simulink model "Copy_of_signal_injection"  (R2023a)
settings: Solver=FixedStepAuto  StartTime=0.0  StopTime=1/(f_fund)/6  FixedStep=1e-7  RelTol=1e-3
InitFcn:
  | f_fund=50;
  | ma=1;
  | fsw=100e3;
settings Model: Creator=enesa  LastModifiedBy=enesa

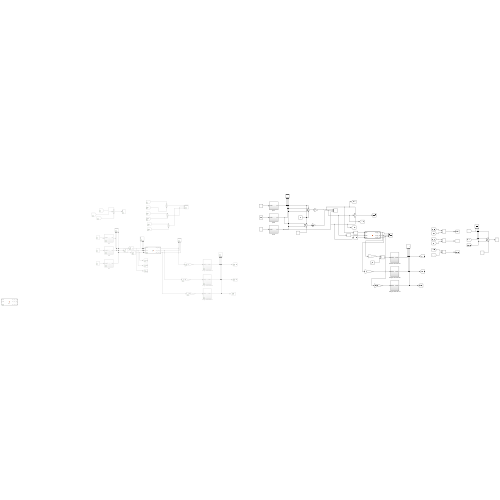
[thumbnail: Simulink's stored preview of the top-level diagram]
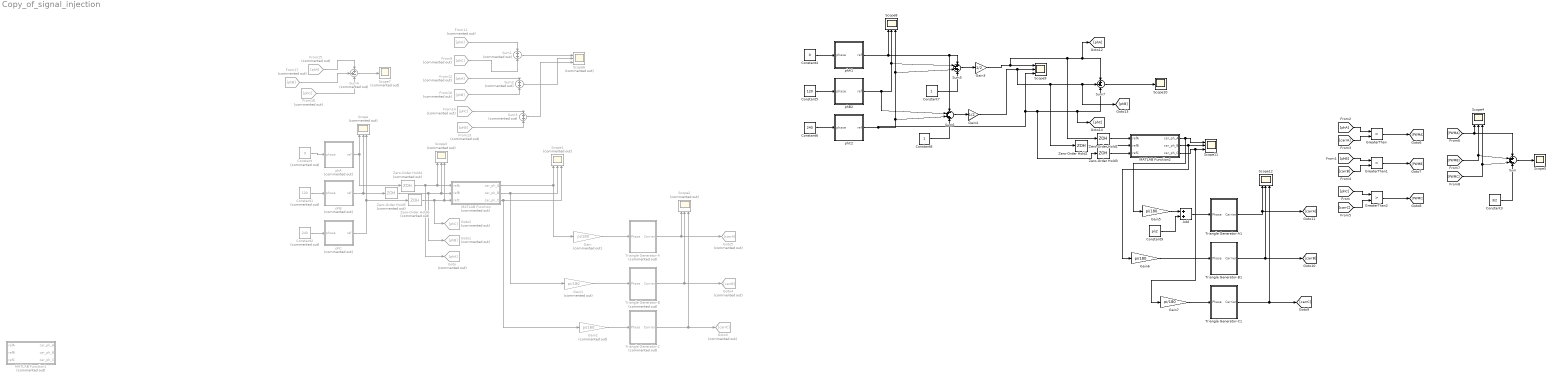
== system Copy_of_signal_injection ==
  Add : Sum
  Constant : Constant  Commented=on  Value=0
  Constant1 : Constant  Commented=on  Value=120
  Constant2 : Constant  Commented=on  Value=240
  Constant3 : Constant  Value=3/2
  Constant4 : Constant  Value=0
  Constant5 : Constant  Value=120
  Constant6 : Constant  Value=240
  Constant7 : Constant
  Constant8 : Constant
  Constant9 : Constant  Value=pi\2
  From10 : From  Commented=on  GotoTag=phB
  From11 : From  Commented=on  GotoTag=phA
  From12 : From  Commented=on  GotoTag=phA
  From13 : From  Commented=on  GotoTag=phB
  From14 : From  Commented=on  GotoTag=phC
  From15 : From  Commented=on  GotoTag=phA
  From16 : From  Commented=on  GotoTag=phC
  From17 : From  Commented=on  GotoTag=phB
  From9 : From  Commented=on  GotoTag=phC
  Gain : Gain  Commented=on  Gain=pi/180
  Gain1 : Gain  Commented=on  Gain=pi/180
  Gain2 : Gain  Commented=on  Gain=pi/180
  Gain3 : Gain  Gain=1/2
  Gain4 : Gain  Gain=1/2
  Gain5 : Gain  Gain=pi/180
  Gain6 : Gain  Gain=pi/180
  Gain7 : Gain  Gain=pi/180
  Goto : Goto  Commented=on  GotoTag=phA
  Goto1 : Goto  Commented=on  GotoTag=phB
  Goto2 : Goto  Commented=on  GotoTag=phC
  Goto3 : Goto  Commented=on  GotoTag=carrC
  Goto4 : Goto  Commented=on  GotoTag=carrB
  Goto5 : Goto  Commented=on  GotoTag=carrA
  GreaterThan : RelationalOperator  Operator=>  OutDataTypeStr=boolean  RndMeth=Simplest  InputSameDT=off
  GreaterThan1 : RelationalOperator  Operator=>  OutDataTypeStr=boolean  RndMeth=Simplest  InputSameDT=off
  GreaterThan2 : RelationalOperator  Operator=>  OutDataTypeStr=boolean  RndMeth=Simplest  InputSameDT=off
  MATLAB Function : MATLAB Function  Commented=on  TreatAsAtomicUnit=on
  MATLAB Function1 : MATLAB Function  Commented=on  TreatAsAtomicUnit=on
  MATLAB Function2 : MATLAB Function  TreatAsAtomicUnit=on
  Scope{,1..3,6} (5 alike) : Scope  Commented=on  NumInputPorts=3
  Scope10 : Scope
  Scope{4,8..9,11..12} (5 alike) : Scope  NumInputPorts=3
  Scope5 : Scope
  Scope7 : Scope  Commented=on
  Sum : Sum  Inputs=+++-
  Sum1 : Sum  Commented=on
  Sum2 : Sum  Commented=on
  Sum3 : Sum  Commented=on
  Sum4 : Sum  Commented=on  Inputs=++-
  Sum5 : Sum  Inputs=+-++
  Sum6 : Sum  Inputs=-+++
  Sum7 : Sum  Inputs=++-
  Triangle Generator-A : Subsystem  Commented=on
  Triangle Generator-A1 : Subsystem
  Triangle Generator-B : Subsystem  Commented=on
  Triangle Generator-B1 : Subsystem
  Triangle Generator-C : Subsystem  Commented=on
  Triangle Generator-C1 : Subsystem
  Zero-Order Hold1 : ZeroOrderHold  SampleTime=20/fsw
  Zero-Order Hold2 : ZeroOrderHold  SampleTime=20/fsw
  Zero-Order Hold3 : ZeroOrderHold  SampleTime=20/fsw
  Zero-Order Hold4 : ZeroOrderHold  Commented=on  SampleTime=20/fsw
  Zero-Order Hold5 : ZeroOrderHold  Commented=on  SampleTime=20/fsw
  Zero-Order Hold6 : ZeroOrderHold  Commented=on  SampleTime=20/fsw
  phA : Subsystem  Commented=on
  phA1 : Subsystem
  phB : Subsystem  Commented=on
  phB2 : Subsystem
  phC : Subsystem  Commented=on
  phC2 : Subsystem
  wires:
  Constant/1 -> phA/1(phase)
  Constant1/1 -> phB/1(phase)
  Constant2/1 -> phC/1(phase)
  phA/1(ref) -> Scope/1, Zero-Order Hold4/1
  phB/1(ref) -> Scope/2, Zero-Order Hold5/1
  phC/1(ref) -> Scope/3, Zero-Order Hold6/1
  MATLAB Function/1(car_ph_A) -> Gain/1, Scope1/1
  MATLAB Function/3(car_ph_C) -> Gain2/1, Scope1/3
  MATLAB Function/2(car_ph_B) -> Gain1/1, Scope1/2
  Triangle Generator-B/1(Carrier) -> Goto4/1, Scope2/2
  Triangle Generator-C/1(Carrier) -> Goto3/1, Scope2/3
  Zero-Order Hold4/1 -> Scope3/1, MATLAB Function/1(refA), Goto/1
  Zero-Order Hold5/1 -> Goto1/1, Scope3/2, MATLAB Function/2(refB)
  Zero-Order Hold6/1 -> Goto2/1, Scope3/3, MATLAB Function/3(refC)
  Triangle Generator-A/1(Carrier) -> Goto5/1, Scope2/1
  [phA] -> GreaterThan/1
  [carrA] -> GreaterThan/2
  [phB] -> GreaterThan1/1
  [carrB] -> GreaterThan1/2
  [phC] -> GreaterThan2/1
  [carrC] -> GreaterThan2/2
  GreaterThan/1 -> [PWMA]
  GreaterThan1/1 -> [PWMB]
  GreaterThan2/1 -> [PWMC]
  [PWMA] -> Sum/1, Scope4/1
  [PWMB] -> Sum/2, Scope4/2
  [PWMC] -> Sum/3, Scope4/3
  Gain/1 -> Triangle Generator-A/1(Phase)
  Gain1/1 -> Triangle Generator-B/1(Phase)
  Gain2/1 -> Triangle Generator-C/1(Phase)
  Sum/1 -> Scope5/1
  Constant3/1 -> Sum/4
  From11/1 -> Sum1/1
  From9/1 -> Sum1/2
  Sum1/1 -> Scope6/1
  From12/1 -> Sum2/1
  From10/1 -> Sum2/2
  Sum2/1 -> Scope6/2
  From13/1 -> Sum3/2
  From14/1 -> Sum3/1
  Sum3/1 -> Scope6/3
  From15/1 -> Sum4/1
  From16/1 -> Sum4/3
  From17/1 -> Sum4/2
  Sum4/1 -> Scope7/1
  Constant6/1 -> phC2/1(phase)
  Constant4/1 -> phA1/1(phase)
  Constant5/1 -> phB2/1(phase)
  Constant7/1 -> Sum5/4
  Sum5/1 -> Gain3/1
  phA1/1(ref) -> Sum6/1, Sum5/1, Scope8/1
  Constant8/1 -> Sum6/4
  Sum6/1 -> Gain4/1
  phB2/1(ref) -> Sum6/2, Sum5/2, Scope8/2
  Gain4/1 -> Zero-Order Hold2/1, [phB], Sum7/2, Scope9/2
  Sum7/1 -> Scope10/1
  MATLAB Function2/1(car_ph_A) -> Gain5/1, Scope11/1
  MATLAB Function2/2(car_ph_B) -> Gain6/1, Scope11/2
  MATLAB Function2/3(car_ph_C) -> Gain7/1, Scope11/3
  phC2/1(ref) -> Zero-Order Hold3/1, [phC], Sum7/3, Scope9/3, Sum6/3, Sum5/3, Scope8/3
  Triangle Generator-A1/1(Carrier) -> [carrA], Scope12/1
  Gain7/1 -> Triangle Generator-C1/1(Phase)
  Gain6/1 -> Triangle Generator-B1/1(Phase)
  Gain3/1 -> [phA], Sum7/1, Zero-Order Hold1/1, Scope9/1
  Triangle Generator-B1/1(Carrier) -> [carrB], Scope12/2
  Triangle Generator-C1/1(Carrier) -> [carrC], Scope12/3
  Zero-Order Hold1/1 -> MATLAB Function2/1(refA)
  Zero-Order Hold2/1 -> MATLAB Function2/2(refB)
  Zero-Order Hold3/1 -> MATLAB Function2/3(refC)
  Gain5/1 -> Add/1
  Constant9/1 -> Add/2
  Add/1 -> Triangle Generator-A1/1(Phase)

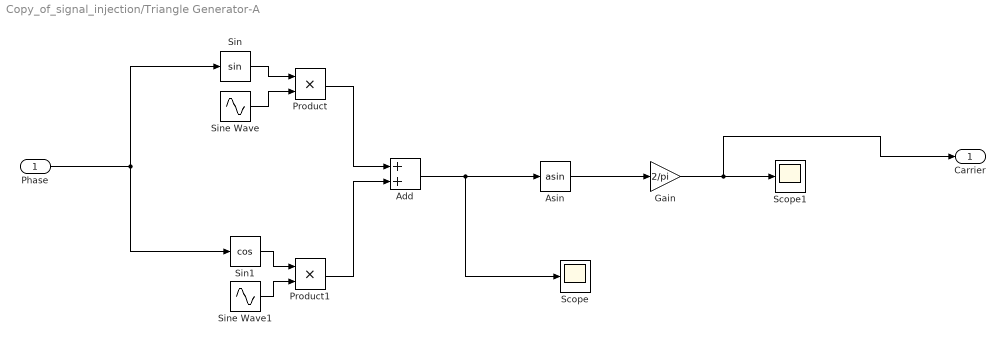
== system Copy_of_signal_injection/Triangle Generator-A ==
  Phase : Inport
  Add : Sum
  Asin : Trigonometry  Operator=asin
  Gain : Gain  Gain=2/pi
  Product : Product
  Product1 : Product
  Scope : Scope
  Scope1 : Scope
  Sin : Trigonometry
  Sin1 : Trigonometry  Operator=cos
  Sine Wave : Sin  Frequency=2*pi*fsw  SampleTime=0
  Sine Wave1 : Sin  Frequency=2*pi*fsw  Phase=-pi/2  SampleTime=0
  Carrier : Outport
  wires:
  Sin/1 -> Product/1
  Sine Wave/1 -> Product/2
  Phase/1 -> Sin/1, Sin1/1
  Product/1 -> Add/1
  Asin/1 -> Gain/1
  Gain/1 -> Carrier/1, Scope1/1
  Sine Wave1/1 -> Product1/2
  Product1/1 -> Add/2
  Add/1 -> Asin/1, Scope/1
  Sin1/1 -> Product1/1

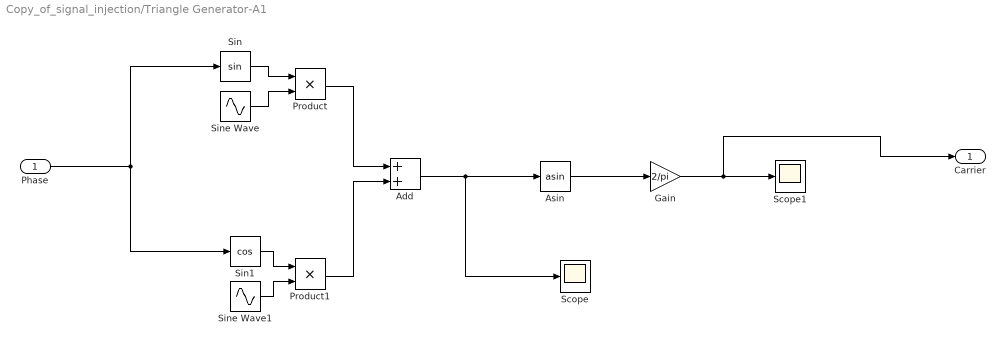
== system Copy_of_signal_injection/Triangle Generator-A1 ==
  Phase : Inport
  Add : Sum
  Asin : Trigonometry  Operator=asin
  Gain : Gain  Gain=2/pi
  Product : Product
  Product1 : Product
  Scope : Scope
  Scope1 : Scope
  Sin : Trigonometry
  Sin1 : Trigonometry  Operator=cos
  Sine Wave : Sin  Frequency=2*pi*fsw  SampleTime=0
  Sine Wave1 : Sin  Frequency=2*pi*fsw  Phase=-pi/2  SampleTime=0
  Carrier : Outport
  wires:
  Sin/1 -> Product/1
  Sine Wave/1 -> Product/2
  Phase/1 -> Sin/1, Sin1/1
  Product/1 -> Add/1
  Asin/1 -> Gain/1
  Gain/1 -> Carrier/1, Scope1/1
  Sine Wave1/1 -> Product1/2
  Product1/1 -> Add/2
  Add/1 -> Asin/1, Scope/1
  Sin1/1 -> Product1/1

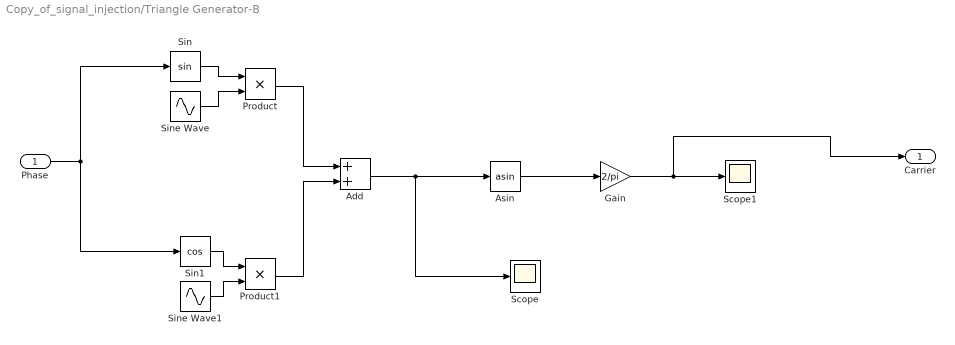
== system Copy_of_signal_injection/Triangle Generator-B ==
  Phase : Inport
  Add : Sum
  Asin : Trigonometry  Operator=asin
  Gain : Gain  Gain=2/pi
  Product : Product
  Product1 : Product
  Scope : Scope
  Scope1 : Scope
  Sin : Trigonometry
  Sin1 : Trigonometry  Operator=cos
  Sine Wave : Sin  Frequency=2*pi*fsw  SampleTime=0
  Sine Wave1 : Sin  Frequency=2*pi*fsw  Phase=-pi/2  SampleTime=0
  Carrier : Outport
  wires:
  Sin/1 -> Product/1
  Sine Wave/1 -> Product/2
  Phase/1 -> Sin1/1, Sin/1
  Product/1 -> Add/1
  Asin/1 -> Gain/1
  Gain/1 -> Carrier/1, Scope1/1
  Sine Wave1/1 -> Product1/2
  Product1/1 -> Add/2
  Add/1 -> Asin/1, Scope/1
  Sin1/1 -> Product1/1

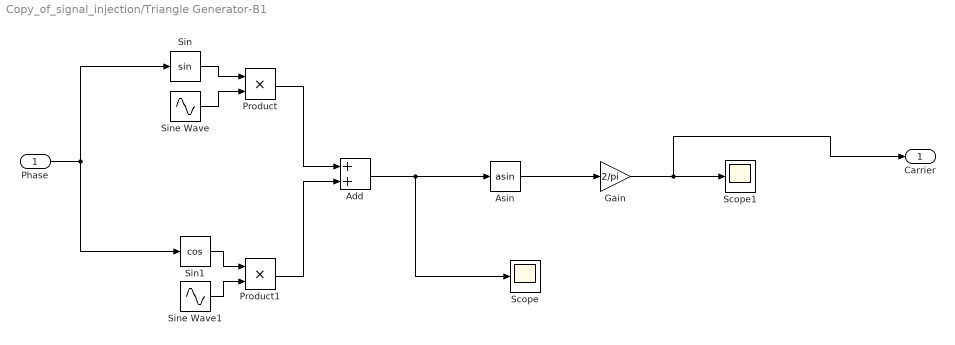
== system Copy_of_signal_injection/Triangle Generator-B1 ==
  Phase : Inport
  Add : Sum
  Asin : Trigonometry  Operator=asin
  Gain : Gain  Gain=2/pi
  Product : Product
  Product1 : Product
  Scope : Scope
  Scope1 : Scope
  Sin : Trigonometry
  Sin1 : Trigonometry  Operator=cos
  Sine Wave : Sin  Frequency=2*pi*fsw  SampleTime=0
  Sine Wave1 : Sin  Frequency=2*pi*fsw  Phase=-pi/2  SampleTime=0
  Carrier : Outport
  wires:
  Sin/1 -> Product/1
  Sine Wave/1 -> Product/2
  Phase/1 -> Sin1/1, Sin/1
  Product/1 -> Add/1
  Asin/1 -> Gain/1
  Gain/1 -> Carrier/1, Scope1/1
  Sine Wave1/1 -> Product1/2
  Product1/1 -> Add/2
  Add/1 -> Asin/1, Scope/1
  Sin1/1 -> Product1/1

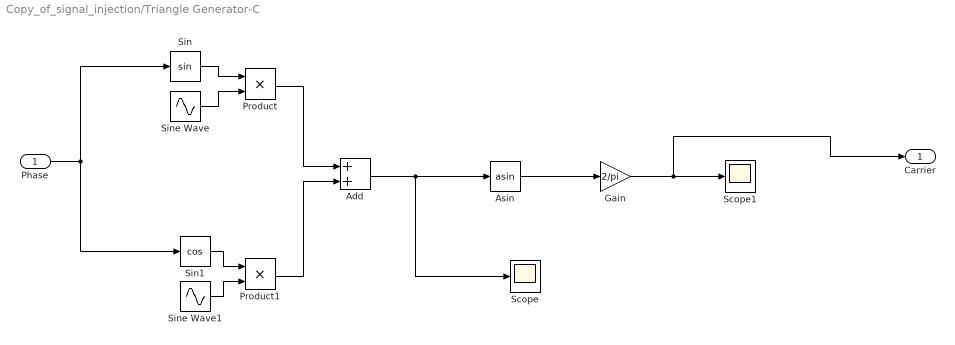
== system Copy_of_signal_injection/Triangle Generator-C ==
  Phase : Inport
  Add : Sum
  Asin : Trigonometry  Operator=asin
  Gain : Gain  Gain=2/pi
  Product : Product
  Product1 : Product
  Scope : Scope
  Scope1 : Scope
  Sin : Trigonometry
  Sin1 : Trigonometry  Operator=cos
  Sine Wave : Sin  Frequency=2*pi*fsw  SampleTime=0
  Sine Wave1 : Sin  Frequency=2*pi*fsw  Phase=-pi/2  SampleTime=0
  Carrier : Outport
  wires:
  Sin/1 -> Product/1
  Sine Wave/1 -> Product/2
  Phase/1 -> Sin1/1, Sin/1
  Product/1 -> Add/1
  Asin/1 -> Gain/1
  Gain/1 -> Carrier/1, Scope1/1
  Sine Wave1/1 -> Product1/2
  Product1/1 -> Add/2
  Add/1 -> Asin/1, Scope/1
  Sin1/1 -> Product1/1

== system Copy_of_signal_injection/Triangle Generator-C1 ==
  Phase : Inport
  Add : Sum
  Asin : Trigonometry  Operator=asin
  Gain : Gain  Gain=2/pi
  Product : Product
  Product1 : Product
  Scope : Scope
  Scope1 : Scope
  Sin : Trigonometry
  Sin1 : Trigonometry  Operator=cos
  Sine Wave : Sin  Frequency=2*pi*fsw  SampleTime=0
  Sine Wave1 : Sin  Frequency=2*pi*fsw  Phase=-pi/2  SampleTime=0
  Carrier : Outport
  wires:
  Sin/1 -> Product/1
  Sine Wave/1 -> Product/2
  Phase/1 -> Sin1/1, Sin/1
  Product/1 -> Add/1
  Asin/1 -> Gain/1
  Gain/1 -> Carrier/1, Scope1/1
  Sine Wave1/1 -> Product1/2
  Product1/1 -> Add/2
  Add/1 -> Asin/1, Scope/1
  Sin1/1 -> Product1/1

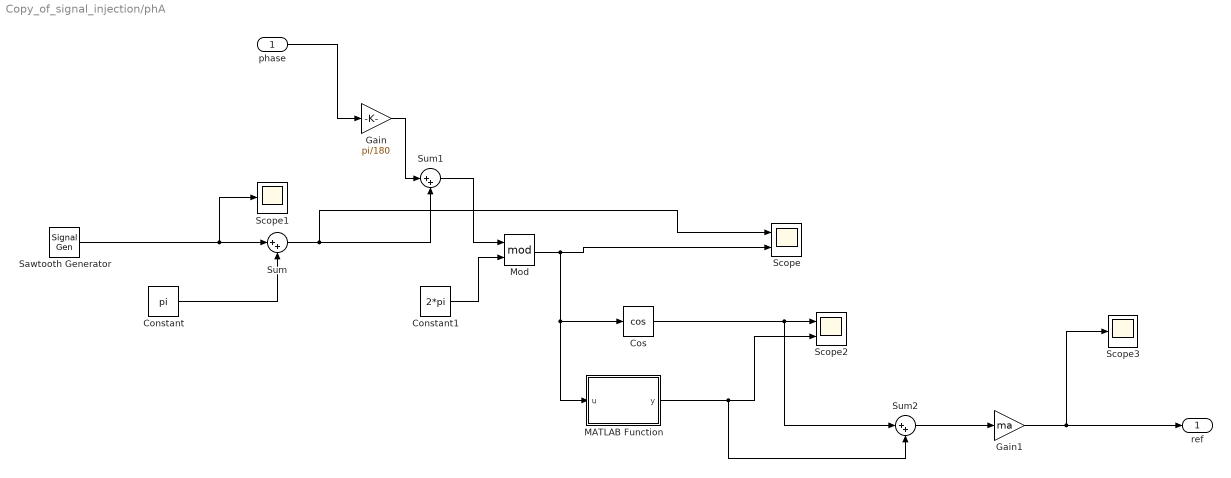
== system Copy_of_signal_injection/phA ==
  phase : Inport
  Constant : Constant  Value=pi
  Constant1 : Constant  Value=2*pi
  Cos : Trigonometry  Operator=cos
  Gain : Gain  Gain=pi/180
  Gain1 : Gain  Gain=ma
  MATLAB Function : MATLAB Function  TreatAsAtomicUnit=on
  Mod : Math  Operator=mod
  Sawtooth Generator : SignalGenerator  WaveForm=sawtooth  Amplitude=pi  Frequency=f_fund
  Scope : Scope  NumInputPorts=2
  Scope1 : Scope
  Scope2 : Scope  NumInputPorts=2
  Scope3 : Scope
  Sum : Sum  Inputs=|++
  Sum1 : Sum  Inputs=|++
  Sum2 : Sum  Inputs=|++
  ref : Outport
  wires:
  phase/1 -> Gain/1
  Sawtooth Generator/1 -> Scope1/1, Sum/1
  Sum/1 -> Sum1/2, Scope/1
  MATLAB Function/1(y) -> Sum2/2, Scope2/2
  Constant/1 -> Sum/2
  Mod/1 -> MATLAB Function/1(u), Cos/1, Scope/2
  Constant1/1 -> Mod/2
  Cos/1 -> Sum2/1, Scope2/1
  Sum1/1 -> Mod/1
  Sum2/1 -> Gain1/1
  Gain/1 -> Sum1/1
  Gain1/1 -> ref/1, Scope3/1

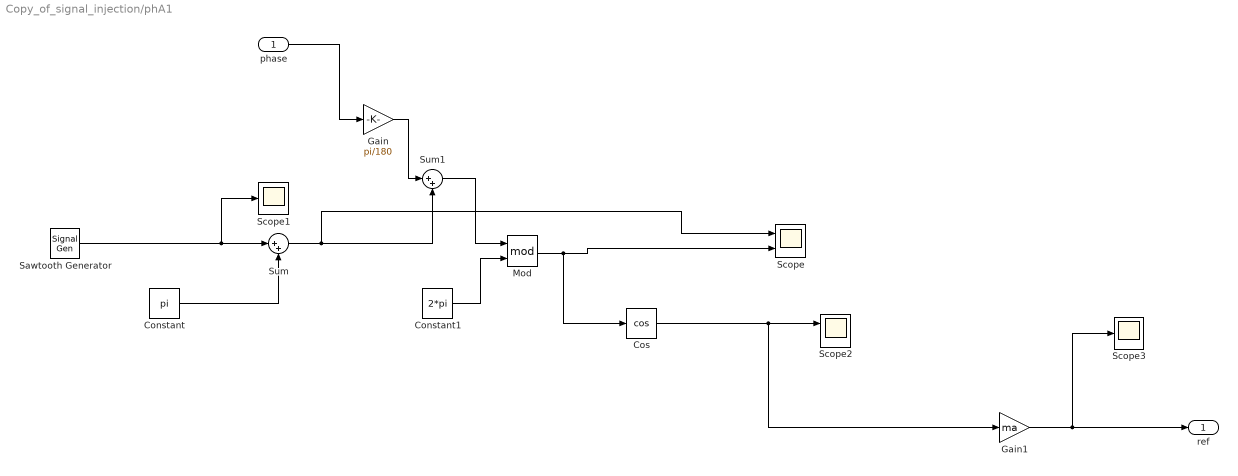
== system Copy_of_signal_injection/phA1 ==
  phase : Inport
  Constant : Constant  Value=pi
  Constant1 : Constant  Value=2*pi
  Cos : Trigonometry  Operator=cos
  Gain : Gain  Gain=pi/180
  Gain1 : Gain  Gain=ma
  Mod : Math  Operator=mod
  Sawtooth Generator : SignalGenerator  WaveForm=sawtooth  Amplitude=pi  Frequency=f_fund
  Scope : Scope  NumInputPorts=2
  Scope1 : Scope
  Scope2 : Scope  NumInputPorts=2
  Scope3 : Scope
  Sum : Sum  Inputs=|++
  Sum1 : Sum  Inputs=|++
  ref : Outport
  wires:
  phase/1 -> Gain/1
  Sawtooth Generator/1 -> Scope1/1, Sum/1
  Sum/1 -> Sum1/2, Scope/1
  Constant/1 -> Sum/2
  Mod/1 -> Cos/1, Scope/2
  Constant1/1 -> Mod/2
  Sum1/1 -> Mod/1
  Cos/1 -> Gain1/1, Scope2/1
  Gain/1 -> Sum1/1
  Gain1/1 -> ref/1, Scope3/1

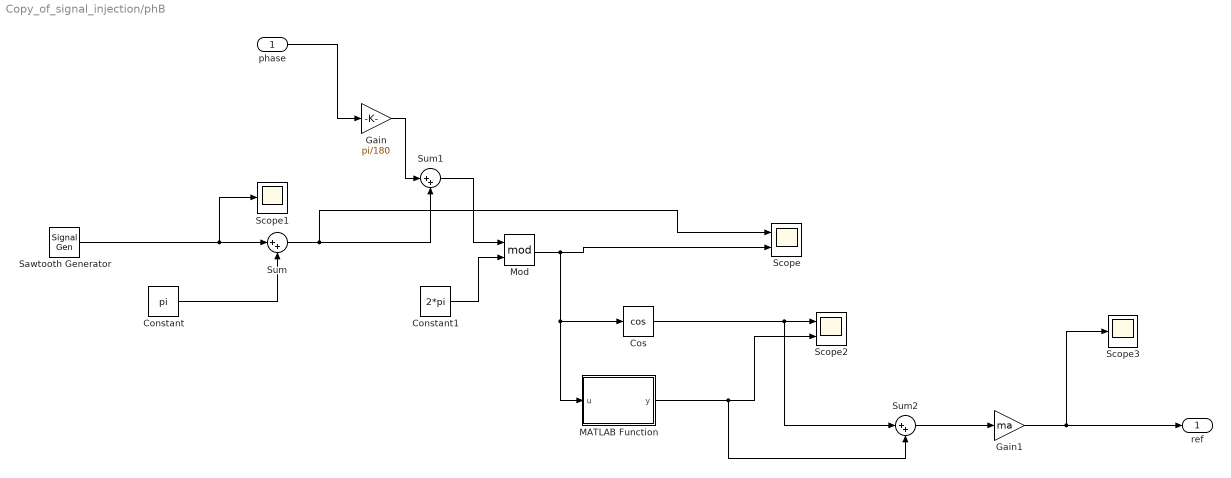
== system Copy_of_signal_injection/phB ==
  phase : Inport
  Constant : Constant  Value=pi
  Constant1 : Constant  Value=2*pi
  Cos : Trigonometry  Operator=cos
  Gain : Gain  Gain=pi/180
  Gain1 : Gain  Gain=ma
  MATLAB Function : MATLAB Function  TreatAsAtomicUnit=on
  Mod : Math  Operator=mod
  Sawtooth Generator : SignalGenerator  WaveForm=sawtooth  Amplitude=pi  Frequency=f_fund
  Scope : Scope  NumInputPorts=2
  Scope1 : Scope
  Scope2 : Scope  NumInputPorts=2
  Scope3 : Scope
  Sum : Sum  Inputs=|++
  Sum1 : Sum  Inputs=|++
  Sum2 : Sum  Inputs=|++
  ref : Outport
  wires:
  phase/1 -> Gain/1
  Sawtooth Generator/1 -> Scope1/1, Sum/1
  Sum/1 -> Sum1/2, Scope/1
  MATLAB Function/1(y) -> Sum2/2, Scope2/2
  Constant/1 -> Sum/2
  Mod/1 -> MATLAB Function/1(u), Cos/1, Scope/2
  Constant1/1 -> Mod/2
  Cos/1 -> Sum2/1, Scope2/1
  Sum1/1 -> Mod/1
  Sum2/1 -> Gain1/1
  Gain/1 -> Sum1/1
  Gain1/1 -> ref/1, Scope3/1

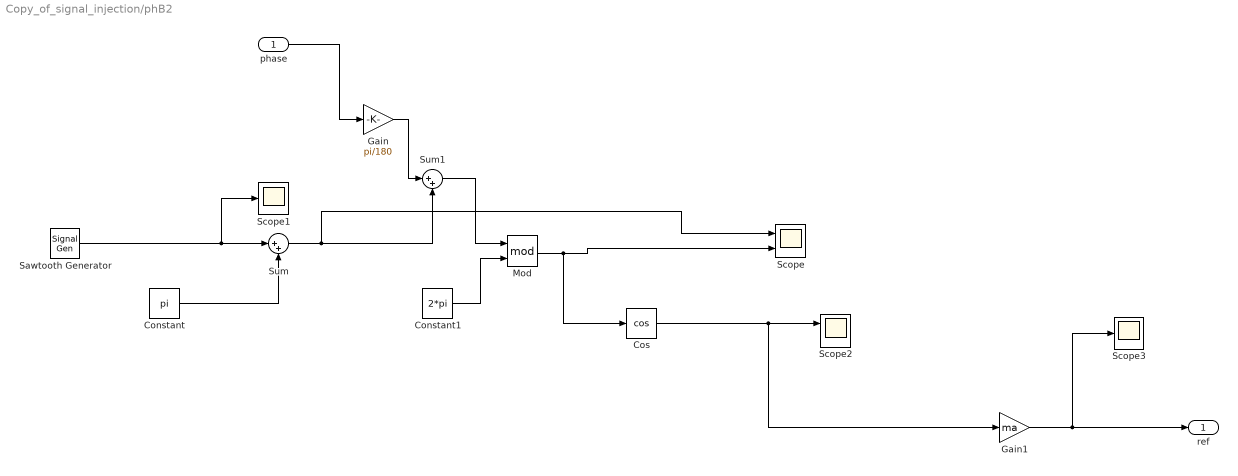
== system Copy_of_signal_injection/phB2 ==
  phase : Inport
  Constant : Constant  Value=pi
  Constant1 : Constant  Value=2*pi
  Cos : Trigonometry  Operator=cos
  Gain : Gain  Gain=pi/180
  Gain1 : Gain  Gain=ma
  Mod : Math  Operator=mod
  Sawtooth Generator : SignalGenerator  WaveForm=sawtooth  Amplitude=pi  Frequency=f_fund
  Scope : Scope  NumInputPorts=2
  Scope1 : Scope
  Scope2 : Scope  NumInputPorts=2
  Scope3 : Scope
  Sum : Sum  Inputs=|++
  Sum1 : Sum  Inputs=|++
  ref : Outport
  wires:
  phase/1 -> Gain/1
  Sawtooth Generator/1 -> Scope1/1, Sum/1
  Sum/1 -> Sum1/2, Scope/1
  Constant/1 -> Sum/2
  Mod/1 -> Cos/1, Scope/2
  Constant1/1 -> Mod/2
  Sum1/1 -> Mod/1
  Cos/1 -> Gain1/1, Scope2/1
  Gain/1 -> Sum1/1
  Gain1/1 -> ref/1, Scope3/1

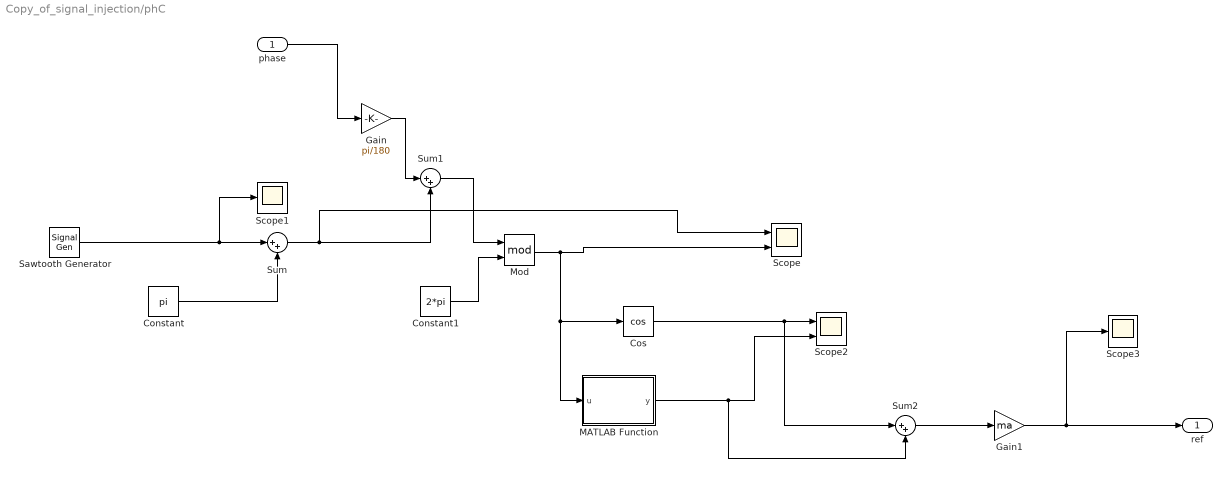
== system Copy_of_signal_injection/phC ==
  phase : Inport
  Constant : Constant  Value=pi
  Constant1 : Constant  Value=2*pi
  Cos : Trigonometry  Operator=cos
  Gain : Gain  Gain=pi/180
  Gain1 : Gain  Gain=ma
  MATLAB Function : MATLAB Function  TreatAsAtomicUnit=on
  Mod : Math  Operator=mod
  Sawtooth Generator : SignalGenerator  WaveForm=sawtooth  Amplitude=pi  Frequency=f_fund
  Scope : Scope  NumInputPorts=2
  Scope1 : Scope
  Scope2 : Scope  NumInputPorts=2
  Scope3 : Scope
  Sum : Sum  Inputs=|++
  Sum1 : Sum  Inputs=|++
  Sum2 : Sum  Inputs=|++
  ref : Outport
  wires:
  phase/1 -> Gain/1
  Sawtooth Generator/1 -> Scope1/1, Sum/1
  Sum/1 -> Sum1/2, Scope/1
  MATLAB Function/1(y) -> Sum2/2, Scope2/2
  Constant/1 -> Sum/2
  Mod/1 -> MATLAB Function/1(u), Cos/1, Scope/2
  Constant1/1 -> Mod/2
  Cos/1 -> Sum2/1, Scope2/1
  Sum1/1 -> Mod/1
  Sum2/1 -> Gain1/1
  Gain/1 -> Sum1/1
  Gain1/1 -> ref/1, Scope3/1

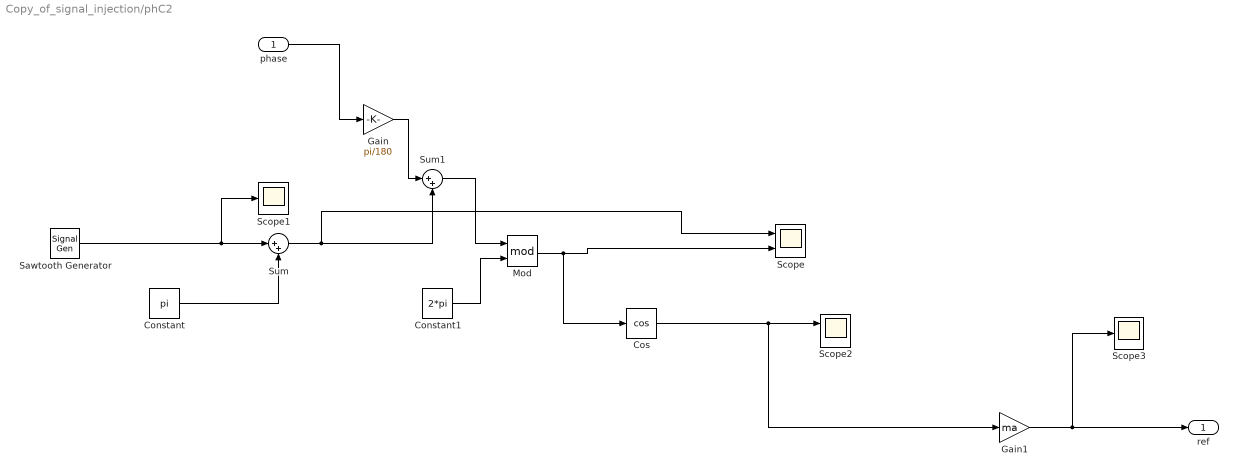
== system Copy_of_signal_injection/phC2 ==
  phase : Inport
  Constant : Constant  Value=pi
  Constant1 : Constant  Value=2*pi
  Cos : Trigonometry  Operator=cos
  Gain : Gain  Gain=pi/180
  Gain1 : Gain  Gain=ma
  Mod : Math  Operator=mod
  Sawtooth Generator : SignalGenerator  WaveForm=sawtooth  Amplitude=pi  Frequency=f_fund
  Scope : Scope  NumInputPorts=2
  Scope1 : Scope
  Scope2 : Scope  NumInputPorts=2
  Scope3 : Scope
  Sum : Sum  Inputs=|++
  Sum1 : Sum  Inputs=|++
  ref : Outport
  wires:
  phase/1 -> Gain/1
  Sawtooth Generator/1 -> Scope1/1, Sum/1
  Sum/1 -> Sum1/2, Scope/1
  Constant/1 -> Sum/2
  Mod/1 -> Cos/1, Scope/2
  Constant1/1 -> Mod/2
  Sum1/1 -> Mod/1
  Cos/1 -> Gain1/1, Scope2/1
  Gain/1 -> Sum1/1
  Gain1/1 -> ref/1, Scope3/1

== matlab function Copy_of_signal_injection/phB/MATLAB Function ==
  data: u input; y output
function y = fcn(u)


if u<=2*pi && u>5*2*pi/6

    y= -(u-5*pi/3)*3/(2*pi)+1/8;

elseif u<=5*2*pi/6 && u>4*2*pi/6

    y= 0;

elseif u<=4*2*pi/6 && u>3*2*pi/6

       y= -(u-4*pi/3)*3/(2*pi)+1/8;

elseif u<=3*2*pi/6 && u>2*2*pi/6

        y= (u-2*pi/3)*3/(2*pi)+1/8;

elseif u<=2*2*pi/6 && u>1*2*pi/6

        y= 0;

elseif u<=2*pi/6 && u>=0

            y= (u-pi/3)*3/(2*pi)+1/8;

else 
    y=0;

end

== matlab function Copy_of_signal_injection/phA/MATLAB Function ==
  data: u input; y output
function y = fcn(u)


if u<=2*pi && u>5*2*pi/6

    y= -(u-5*pi/3)*3/(2*pi)+1/8;

elseif u<=5*2*pi/6 && u>4*2*pi/6

    y= 0;

elseif u<=4*2*pi/6 && u>3*2*pi/6

       y= -(u-4*pi/3)*3/(2*pi)+1/8;

elseif u<=3*2*pi/6 && u>2*2*pi/6

        y= (u-2*pi/3)*3/(2*pi)+1/8;

elseif u<=2*2*pi/6 && u>1*2*pi/6

        y= 0;

elseif u<=2*pi/6 && u>=0

            y= (u-pi/3)*3/(2*pi)+1/8;

else 
    y=0;

end

== matlab function Copy_of_signal_injection/phC/MATLAB Function ==
  data: u input; y output
function y = fcn(u)


if u<=2*pi && u>5*2*pi/6

    y= -(u-5*pi/3)*3/(2*pi)+1/8;

elseif u<=5*2*pi/6 && u>4*2*pi/6

    y= 0;

elseif u<=4*2*pi/6 && u>3*2*pi/6

       y= -(u-4*pi/3)*3/(2*pi)+1/8;

elseif u<=3*2*pi/6 && u>2*2*pi/6

        y= (u-2*pi/3)*3/(2*pi)+1/8;

elseif u<=2*2*pi/6 && u>1*2*pi/6

        y= 0;

elseif u<=2*pi/6 && u>=0

            y= (u-pi/3)*3/(2*pi)+1/8;

else 
    y=0;

end

== matlab function Copy_of_signal_injection/MATLAB Function ==
  data: refA input; car_ph_A output; refB input; refC input; car_ph_B output; car_ph_C output
function [car_ph_A, car_ph_B, car_ph_C]= fcn(refA, refB, refC)

refA2=(1+refA)/2;
refB2=(1+refB)/2;
refC2=(1+refC)/2,

if refA2>=refB2 && refA2>=refC2

if refB2>=refC2 
car_ph_B=0;
car_ph_C=((refA2-refC2)/2)*360;
car_ph_A=((refA2+refB2-2*refC2)/2)*360;
else
car_ph_C=0;
car_ph_B=((refA2-refB2)/2)*360;
car_ph_A=((refA2+refC2-2*refB2)/2)*360;
end

elseif refB2>=refA2 && refB2>=refC2

if refA2>=refC2 
car_ph_A=0;
car_ph_C=((refB2-refC2)/2)*360;
car_ph_B=((refA2+refB2-2*refC2)/2)*360;
else
car_ph_C=0;
car_ph_A=((refB2-refA2)/2)*360;
car_ph_B=((refB2+refC2-2*refA2)/2)*360;
end

elseif refC2>=refA2 && refC2>=refB2

if refA2>=refB2 
car_ph_A=0;
car_ph_B=((refC2-refB2)/2)*360;
car_ph_C=((refA2+refC2-2*refB2)/2)*360;

else
car_ph_B=0;
car_ph_A=((refC2-refA2)/2)*360;
car_ph_C=((refB2+refC2-2*refA2)/2)*360;

end


else

car_ph_A=0;
car_ph_B=0;
car_ph_C=0;

end





end

== matlab function Copy_of_signal_injection/MATLAB Function1 ==
  data: refA input; car_ph_A output; refB input; refC input; car_ph_B output; car_ph_C output
function [car_ph_A, car_ph_B, car_ph_C]= fcn(refA, refB, refC)

refA2=(1+refA)/2;
refB2=(1+refB)/2;
refC2=(1+refC)/2,

if refA2>=refB2 && refA2>=refC2

car_ph_A=0;

if refB2>=refC2 

car_ph_C=((refA2-refC2)/2)*360;
car_ph_B=((refA2+refB2-2*refC2)/2)*360;

else

car_ph_B=((refA2-refB2)/2)*360;
car_ph_C=((refA2+refC2-2*refB2)/2)*360;

end

elseif refB2>=refA2 && refB2>=refC2

car_ph_B=0;

if refA2>=refC2 

car_ph_C=((refB2-refC2)/2)*360;
car_ph_A=((refA2+refB2-2*refC2)/2)*360;

else

car_ph_A=((refB2-refA2)/2)*360;
car_ph_C=((refB2+refC2-2*refA2)/2)*360;

end

elseif refC2>=refA2 && refC2>=refB2

car_ph_C=0;

if refA2>=refB2 

car_ph_B=((refC2-refB2)/2)*360;
car_ph_A=((refA2+refC2-2*refB2)/2)*360;

else

car_ph_A=((refC2-refA2)/2)*360;
car_ph_B=((refB2+refC2-2*refA2)/2)*360;

end


else

car_ph_A=0;
car_ph_B=0;
car_ph_C=0;

end





end

== matlab function Copy_of_signal_injection/MATLAB Function2 ==
  data: refA input; car_ph_A output; refB input; refC input; car_ph_B output; car_ph_C output
function [car_ph_A, car_ph_B, car_ph_C]= fcn(refA, refB, refC)

refA2=(1+refA)/2;
refB2=(1+refB)/2;
refC2=(1+refC)/2,

car_ph_A=0;
car_ph_C=360*(refA2+refC2)/2;
car_ph_B=360*(refA2+refB2-2*refC2)/2;


end
